simulink model "LaneGuidance"  (R2022b)
settings: Solver=FixedStepAuto  StartTime=0.0  StopTime=10.0  FixedStep=1/10  RelTol=1e-3
model workspace (MAT data in the model file):
  HazardLightsOFF = Simulink.Parameter
  HazardLightsOFF.Value = 0
  HazardLightsOFF.DataType = 'auto'
  HazardLightsOFF.Complexity = 'real'
  HazardLightsOFF.Dimensions = [1 1]
  HazardLightsON = Simulink.Parameter
  HazardLightsON.Value = 1
  HazardLightsON.DataType = 'auto'
  HazardLightsON.Complexity = 'real'
  HazardLightsON.Dimensions = [1 1]
  SafeDistanceThreshold = Simulink.Parameter
  SafeDistanceThreshold.Value = 0.1
  SafeDistanceThreshold.DataType = 'auto'
  SafeDistanceThreshold.Complexity = 'real'
  SafeDistanceThreshold.Dimensions = [1 1]
settings Model: Creator=The MathWorks, Inc.  LastModifiedBy=The MathWorks, Inc.
settings SolverCC: AlgebraicLoopSolver=TrustRegion
settings DataIOCC: ReturnWorkspaceOutputs=off
settings OptimizationCC: DefaultParameterBehavior=Inlined  EnhancedBackFolding=on  PassReuseOutputArgsAs=Individual arguments  ZeroExternalMemoryAtStartup=off  ZeroInternalMemoryAtStartup=off  OptimizeBlockOrder=speed  DifferentSizesBufferReuse=on  OptimizationCustomize=off  EfficientTunableParamExpr=on
settings DebuggingCC: ParameterTunabilityLossMsg=error  UnconnectedInputMsg=warning  UnconnectedOutputMsg=warning  UnconnectedLineMsg=warning  SFMachineParentedDataDiag=warning  ArithmeticOperatorsInVariantConditions=warning
settings HardwareCC: ProdBitPerLong=64  ProdHWDeviceType=Intel->x86-64 (Linux 64)
settings ModelReferenceCC: EnableRefExpFcnMdlSchedulingChecks=on
settings SFSimCC: SimUseLocalCustomCode=off  MATLABDynamicMemAlloc=off  CustomCodeUndefinedFunction=UseInterfaceOnly
settings RTWCC: Description=Embedded Coder  SystemTargetFile=ert.tlc  PackageName=mApp.zip  TemplateMakefile=ert_default_tmf  GenerateReport=on  RTWUseLocalCustomCode=off  IncludeHyperlinkInReport=on  LaunchReport=on  GenerateTraceInfo=on  GenerateTraceReport=on  GenerateTraceReportSl=on  GenerateTraceReportSf=on  GenerateTraceReportEml=on
settings CodeAppCC: ForceParamTrailComments=on  IgnoreCustomStorageClasses=off  OperatorAnnotations=on  SimulinkDataObjDesc=on  SFDataObjDesc=on  InsertBlockDesc=on
settings ERTTargetCC: TargetLangStandard=C99 (ISO)  GenerateSampleERTMain=on  InlinedParameterPlacement=NonHierarchical  ERTCustomFileTemplate=example_file_process.tlc

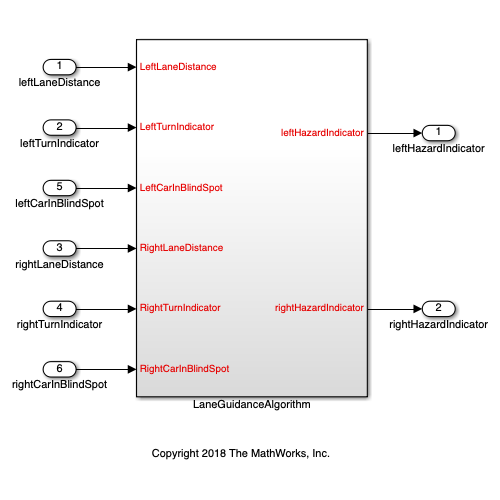
[thumbnail: Simulink's stored preview of the top-level diagram]
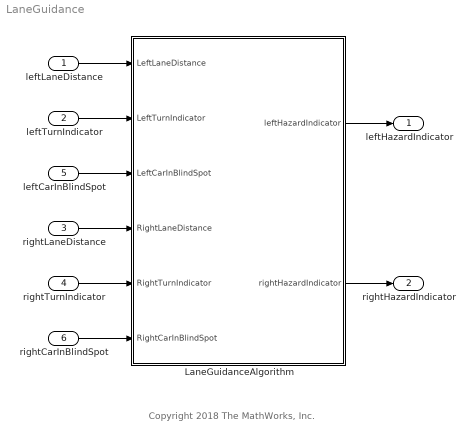
== system LaneGuidance ==
  note: Copyright 2018 The MathWorks, Inc.
  leftLaneDistance : Inport  OutDataTypeStr=double  PortDimensions=1
  leftTurnIndicator : Inport  Port=2  OutDataTypeStr=double  PortDimensions=1
  rightLaneDistance : Inport  Port=3  OutDataTypeStr=double  PortDimensions=1
  rightTurnIndicator : Inport  Port=4  OutDataTypeStr=double  PortDimensions=1
  leftCarInBlindSpot : Inport  Port=5  OutDataTypeStr=double  PortDimensions=1
  rightCarInBlindSpot : Inport  Port=6  OutDataTypeStr=double  PortDimensions=1
  LaneGuidanceAlgorithm : Subsystem
  leftHazardIndicator : Outport  OutDataTypeStr=double  PortDimensions=1  VectorParamsAs1DForOutWhenUnconnected=off
  rightHazardIndicator : Outport  Port=2  OutDataTypeStr=double  PortDimensions=1  VectorParamsAs1DForOutWhenUnconnected=off
  wires:
  leftLaneDistance/1 -> LaneGuidanceAlgorithm/1(LeftLaneDistance)
  rightLaneDistance/1 -> LaneGuidanceAlgorithm/4(RightLaneDistance)
  LaneGuidanceAlgorithm/1(leftHazardIndicator) -> leftHazardIndicator/1
  rightTurnIndicator/1 -> LaneGuidanceAlgorithm/5(RightTurnIndicator)
  leftTurnIndicator/1 -> LaneGuidanceAlgorithm/2(LeftTurnIndicator)
  leftCarInBlindSpot/1 -> LaneGuidanceAlgorithm/3(LeftCarInBlindSpot)
  rightCarInBlindSpot/1 -> LaneGuidanceAlgorithm/6(RightCarInBlindSpot)
  LaneGuidanceAlgorithm/2(rightHazardIndicator) -> rightHazardIndicator/1

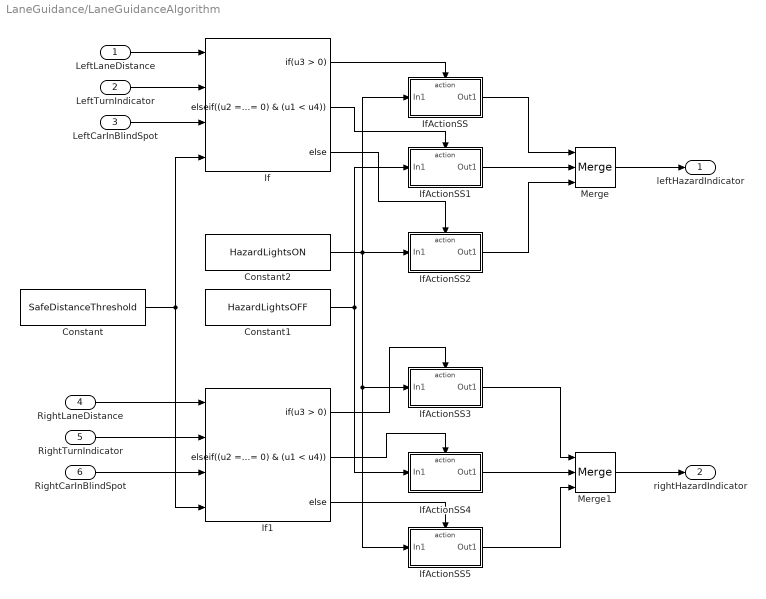
== system LaneGuidance/LaneGuidanceAlgorithm ==
  LeftLaneDistance : Inport
  LeftTurnIndicator : Inport  Port=2
  LeftCarInBlindSpot : Inport  Port=3
  RightLaneDistance : Inport  Port=4
  RightTurnIndicator : Inport  Port=5
  RightCarInBlindSpot : Inport  Port=6
  Constant : Constant  Value=SafeDistanceThreshold
  Constant1 : Constant  Value=HazardLightsOFF
  Constant2 : Constant  Value=HazardLightsON
  If : If  NumInputs=4  IfExpression=u3 > 0  ElseIfExpressions=(u2 == 0) & (u1 < u4)
  If1 : If  NumInputs=4  IfExpression=u3 > 0  ElseIfExpressions=(u2 == 0) & (u1 < u4)
  IfActionSS : Subsystem  TreatAsAtomicUnit=on
  IfActionSS1 : Subsystem  TreatAsAtomicUnit=on
  IfActionSS2 : Subsystem  TreatAsAtomicUnit=on
  IfActionSS3 : Subsystem  TreatAsAtomicUnit=on
  IfActionSS4 : Subsystem  TreatAsAtomicUnit=on
  IfActionSS5 : Subsystem  TreatAsAtomicUnit=on
  Merge : Merge  Inputs=3
  Merge1 : Merge  Inputs=3
  leftHazardIndicator : Outport  VectorParamsAs1DForOutWhenUnconnected=off
  rightHazardIndicator : Outport  Port=2  VectorParamsAs1DForOutWhenUnconnected=off
  wires:
  Merge/1 -> leftHazardIndicator/1
  If/3 -> IfActionSS2/Action
  Constant/1 -> If/4, If1/4
  LeftCarInBlindSpot/1 -> If/3
  LeftTurnIndicator/1 -> If/2
  LeftLaneDistance/1 -> If/1
  IfActionSS2/1(Out1) -> Merge/3
  IfActionSS1/1(Out1) -> Merge/2
  IfActionSS/1(Out1) -> Merge/1
  If/1 -> IfActionSS/Action
  If/2 -> IfActionSS1/Action
  Constant2/1 -> IfActionSS5/1(In1), IfActionSS3/1(In1), IfActionSS/1(In1), IfActionSS2/1(In1)
  Constant1/1 -> IfActionSS4/1(In1), IfActionSS1/1(In1)
  If1/2 -> IfActionSS4/Action
  If1/1 -> IfActionSS3/Action
  IfActionSS3/1(Out1) -> Merge1/1
  IfActionSS4/1(Out1) -> Merge1/2
  IfActionSS5/1(Out1) -> Merge1/3
  If1/3 -> IfActionSS5/Action
  Merge1/1 -> rightHazardIndicator/1
  RightLaneDistance/1 -> If1/1
  RightTurnIndicator/1 -> If1/2
  RightCarInBlindSpot/1 -> If1/3

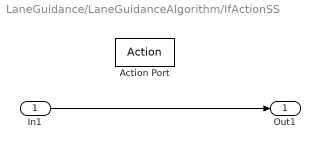
== system LaneGuidance/LaneGuidanceAlgorithm/IfActionSS ==
  In1 : Inport
  Action Port : ActionPort  ActionPortLabel=if(u3 > 0)
  Out1 : Outport  VectorParamsAs1DForOutWhenUnconnected=off
  wires:
  In1/1 -> Out1/1

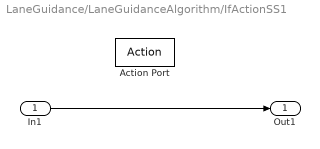
== system LaneGuidance/LaneGuidanceAlgorithm/IfActionSS1 ==
  In1 : Inport
  Action Port : ActionPort  ActionPortLabel=elseif((u2 == 0) & (u1 < u4))
  Out1 : Outport  VectorParamsAs1DForOutWhenUnconnected=off
  wires:
  In1/1 -> Out1/1

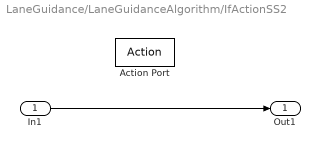
== system LaneGuidance/LaneGuidanceAlgorithm/IfActionSS2 ==
  In1 : Inport
  Action Port : ActionPort  ActionPortLabel=else
  Out1 : Outport  VectorParamsAs1DForOutWhenUnconnected=off
  wires:
  In1/1 -> Out1/1

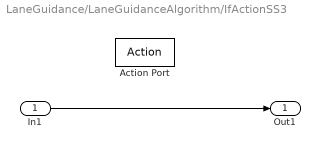
== system LaneGuidance/LaneGuidanceAlgorithm/IfActionSS3 ==
  In1 : Inport
  Action Port : ActionPort  ActionPortLabel=if(u3 > 0)
  Out1 : Outport  VectorParamsAs1DForOutWhenUnconnected=off
  wires:
  In1/1 -> Out1/1

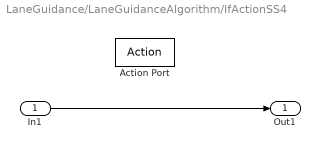
== system LaneGuidance/LaneGuidanceAlgorithm/IfActionSS4 ==
  In1 : Inport
  Action Port : ActionPort  ActionPortLabel=elseif((u2 == 0) & (u1 < u4))
  Out1 : Outport  VectorParamsAs1DForOutWhenUnconnected=off
  wires:
  In1/1 -> Out1/1

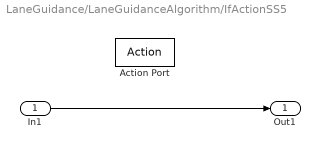
== system LaneGuidance/LaneGuidanceAlgorithm/IfActionSS5 ==
  In1 : Inport
  Action Port : ActionPort  ActionPortLabel=else
  Out1 : Outport  VectorParamsAs1DForOutWhenUnconnected=off
  wires:
  In1/1 -> Out1/1
